simulink model "homework_2_2_29"  (R2021b)
settings: Solver=VariableStepAuto  StartTime=0.0  StopTime=10.0  RelTol=1e-3
settings Model: Creator=DELL  LastModifiedBy=DELL

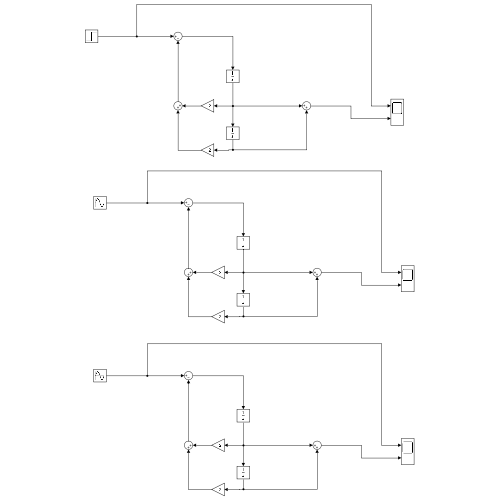
[thumbnail: Simulink's stored preview of the top-level diagram]
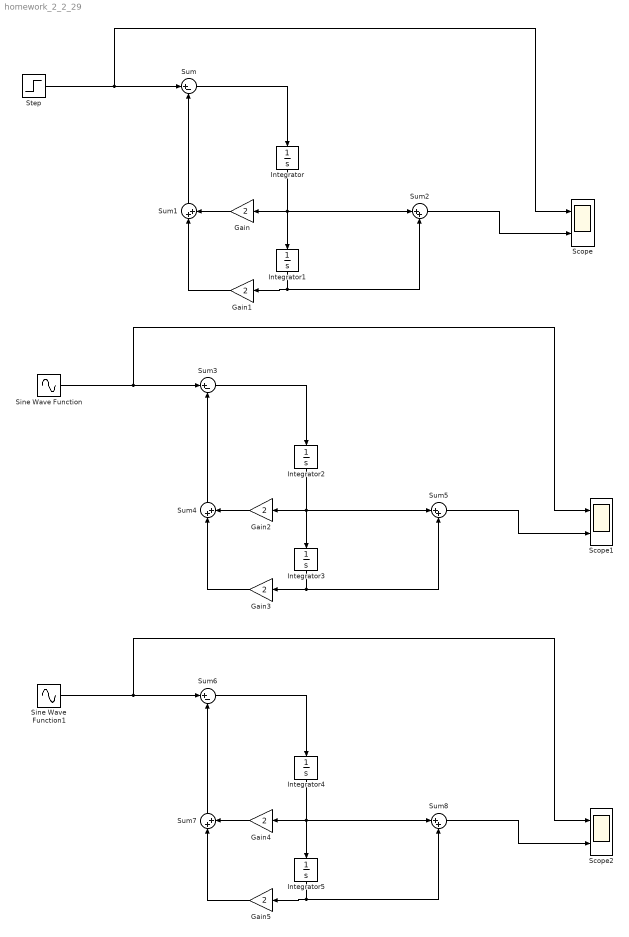
== system homework_2_2_29 ==
  Gain{,1..5} (6 alike) : Gain  Gain=2
  Integrator{,1..5} (6 alike) : Integrator
  Scope : Scope  NumInputPorts=2
  Scope1 : Scope  NumInputPorts=2
  Scope2 : Scope  NumInputPorts=2
  Sine Wave Function : Sin  Frequency=3  SampleTime=0
  Sine Wave Function1 : Sin  SampleTime=0
  Step : Step  SampleTime=0
  Sum : Sum  Inputs=|+-
  Sum{1..2,4..5,7..8} (6 alike) : Sum  Inputs=|++
  Sum3 : Sum  Inputs=|+-
  Sum6 : Sum  Inputs=|+-
  wires:
  Sum/1 -> Integrator/1
  Integrator/1 -> Integrator1/1, Gain/1, Sum2/1
  Sum1/1 -> Sum/2
  Step/1 -> Scope/1, Sum/1
  Integrator1/1 -> Gain1/1, Sum2/2
  Sum2/1 -> Scope/2
  Gain/1 -> Sum1/2
  Gain1/1 -> Sum1/1
  Sum5/1 -> Scope1/2
  Sine Wave Function/1 -> Scope1/1, Sum3/1
  Sum4/1 -> Sum3/2
  Integrator3/1 -> Gain3/1, Sum5/2
  Gain2/1 -> Sum4/2
  Integrator2/1 -> Integrator3/1, Gain2/1, Sum5/1
  Sum3/1 -> Integrator2/1
  Gain3/1 -> Sum4/1
  Sine Wave Function1/1 -> Scope2/1, Sum6/1
  Gain5/1 -> Sum7/1
  Sum6/1 -> Integrator4/1
  Integrator4/1 -> Integrator5/1, Gain4/1, Sum8/1
  Gain4/1 -> Sum7/2
  Integrator5/1 -> Gain5/1, Sum8/2
  Sum8/1 -> Scope2/2
  Sum7/1 -> Sum6/2
